simulink model "Exercise18real"  (Simulink 7.2)
settings: Solver=ode45  StartTime=0.0  StopTime=10.0  RelTol=1e-3
libraries: simulink x2
settings Model: Creator=Inderjot  LastModifiedBy=Inderjot

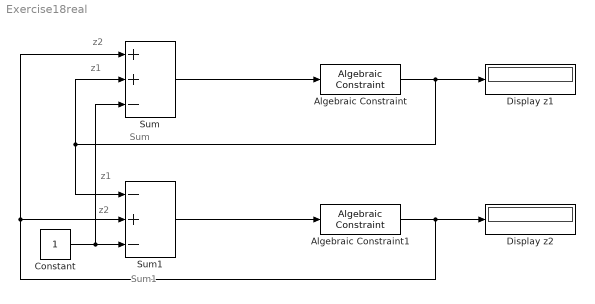
== system Exercise18real ==
  note: z2
  note: z1
  note: z1
  note: z2
  note: Sum1
  note: Sum
  Algebraic Constraint : simulink/Math Operations/Algebraic Constraint  SystemSampleTime=-1  z0=0
  Algebraic Constraint1 : simulink/Math Operations/Algebraic Constraint  SystemSampleTime=-1  z0=0
  Constant : Constant  OutDataType=sfix(16)  OutScaling=2^0
  Display z1 : Display
  Display z2 : Display
  Sum : Sum  Inputs=++-  OutDataType=sfix(16)  OutScaling=2^0
  Sum1 : Sum  Inputs=-+-  OutDataType=sfix(16)  OutScaling=2^0
  wires:
  Sum/1 -> Algebraic Constraint/1
  Sum1/1 -> Algebraic Constraint1/1
  Algebraic Constraint/1 -> Display z1/1, Sum/2, Sum1/1
  Algebraic Constraint1/1 -> Display z2/1, Sum1/2, Sum/1
  Constant/1 -> Sum1/3, Sum/3
